simulink model "RightCameraAgent"  (Simulink 6.2)
settings: Solver=ode45  StartTime=0.0  StopTime=10.0  RelTol=1e-3
settings Model: LastModifiedBy=suarezjl
settings DataIOCC: SignalLoggingName=sigsOut
settings HardwareCC: TargetUnknown=on

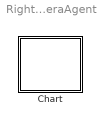
== system RightCameraAgent ==
  Chart : Stateflow chart

== stateflow chart Chart ==
  state Initial
    \\Sally\CogDemo\HeadModule\RightCameraAgent\FrameGrabber.Initialize()
    \\Sally\CogDemo\HeadModule\RightCameraAgent\FrameGrabber.ObtainImage()
    \\Sally\CogDemo\HeadModule\RightCameraAgent\FrameGrabber.ObtainImage()
    \\Sally\CogDemo\HeadModule\RightCameraAgent\ColorBarney.Initialize()
    \\Sally\CogDemo\HeadModule\RightCameraAgent\ColorBarney.LoadColorModel()
    \\Sally\CogDemo\HeadModule\RightCameraAgent\ColorBlue.Initialize()
    \\Sally\CogDemo\HeadModule\RightCameraAgent\ColorBlue.LoadColorModel()
    \\Sally\CogDemo\HeadModule\RightCameraAgent\ColorRed.Initialize()
    \\Sally\CogDemo\HeadModule\RightCameraAgent\ColorRed.LoadColorModel()
  state Segmentation
    \\Sally\CogDemo\HeadModule\RightCameraAgent\FrameGrabber.ObtainImage()
    \\Sally\CogDemo\HeadModule\RightCameraAgent\ColorBarney.DoSegment()
    \\Sally\CogDemo\HeadModule\RightCameraAgent\ColorBlue.DoSegment()
    \\Sally\CogDemo\HeadModule\RightCameraAgent\ColorRed.DoSegment()
  (default) -> Initial : Start
  Initial -> Segmentation : Always
  Segmentation -> Segmentation : Always
